simulink model "Main_C0_C3"  (R2023a)
settings: Solver=ode15s  StartTime=0.0  StopTime=1  RelTol=1e-3
model workspace (MAT data in the model file):
  C_IVD = 0.05
  E_IVD1 = 2.1
  E_IVD2 = 2.2
  E_IVD3 = 1.1
  E_IVD4 = 1.7
  E_IVD5 = 3.2
  IVD1 : object (value not decoded)
  IVD2 : object (value not decoded)
  IVD3 : object (value not decoded)
  IVD4 : object (value not decoded)
  IVD5 : object (value not decoded)
  eo_color = [1 0 0]
  io_color = [0 1 0]
  longissimus_color = [1 0 1]
  multifidus_color = [0 1 1]
  muscle_radius = 1
  psoas_color = [0 0 1]
  ra_color = [1 1 0.5]
symbols that are objects in the model workspace (value not decoded): IVD1, IVD2, IVD3, IVD4, IVD5
undefined symbols (not defined in the file or in its folder): AbdFlex, E_TLFflex, IAP_activation_AbdFlex, IAP_Pa, LeftAbdominalMuscleForce, LeftBackMuscleForce, LeftTransverse1MuscleForce, LeftTransverse2MuscleForce, RightAbdominalMuscleForce, RightBackMuscleForce, RightTransverse1MuscleForce, RightTransverse2MuscleForce, TLFflex2, X, Y, Z
libraries: nesl_utility x1235, sm_lib x960, fl_lib x6, simulink_extras x2
(part 8 of 37)

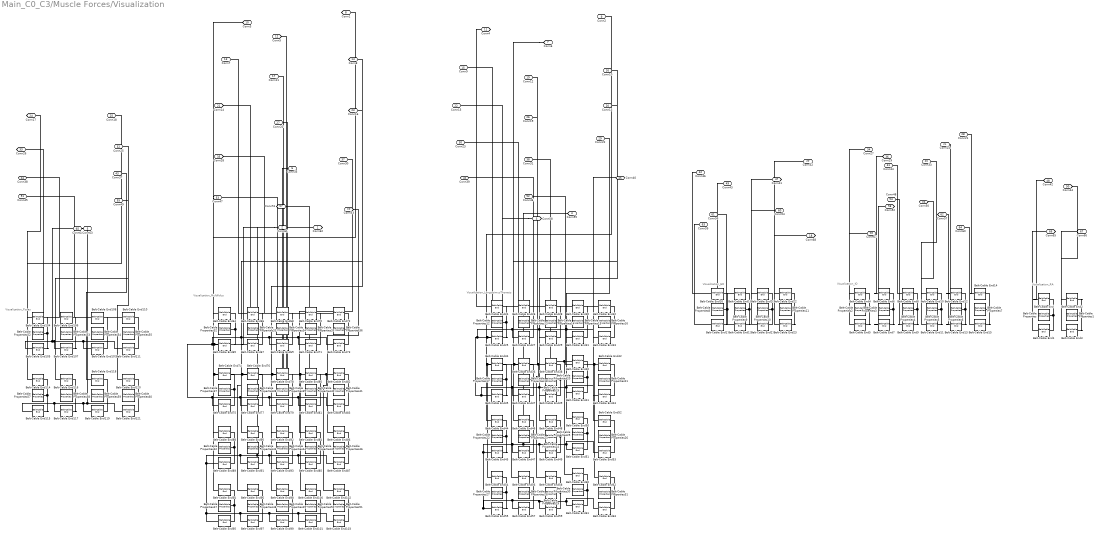
== system Main_C0_C3/Muscle Forces/Visualization ==
  note: Visualization_RA
  note: Visualization_IO
  note: Visualization_EO
  note: Visualization_LongissimusThoracis
  note: Visualization_Multifidus
  note: Visualization_Psoas
  Belt-Cable Properties : sm_lib/Belts and Cables/Belt-Cable Properties  DrumBeltCableAlignment=Unrestricted  GraphicType=PitchLine  GraphicVisPropType=SimpleVisualProperties  GraphicDiffuseColor=[0.302 0.7451 0.9333]  GraphicSpecularColor=[0.5 0.5 0.5 1.0]  GraphicAmbientColor=[0.15 0.15 0.15 1.0]  GraphicEmissiveColor=[0.0 0.0 0.0 1.0]  GraphicShininess=75  GraphicOpacity=1.0
  Belt-Cable Properties1 : sm_lib/Belts and Cables/Belt-Cable Properties  DrumBeltCableAlignment=Unrestricted  GraphicType=PitchLine  GraphicVisPropType=SimpleVisualProperties  GraphicDiffuseColor=[0.302 0.7451 0.9333]  GraphicSpecularColor=[0.5 0.5 0.5 1.0]  GraphicAmbientColor=[0.15 0.15 0.15 1.0]  GraphicEmissiveColor=[0.0 0.0 0.0 1.0]  GraphicShininess=75  GraphicOpacity=1.0
  Belt-Cable Properties{8..11} (4 alike) : sm_lib/Belts and Cables/Belt-Cable Properties  DrumBeltCableAlignment=Unrestricted  GraphicType=PitchLine  GraphicVisPropType=SimpleVisualProperties  GraphicDiffuseColor=[0.851 0.3255 0.09804]  GraphicSpecularColor=[0.5 0.5 0.5 1.0]  GraphicAmbientColor=[0.15 0.15 0.15 1.0]  GraphicEmissiveColor=[0.0 0.0 0.0 1.0]  GraphicShininess=75  GraphicOpacity=1.0
  Belt-Cable Properties{12..31} (20 alike) : sm_lib/Belts and Cables/Belt-Cable Properties  DrumBeltCableAlignment=Unrestricted  GraphicType=PitchLine  GraphicVisPropType=SimpleVisualProperties  GraphicDiffuseColor=[0 0 1]  GraphicSpecularColor=[0.5 0.5 0.5 1.0]  GraphicAmbientColor=[0.15 0.15 0.15 1.0]  GraphicEmissiveColor=[0.0 0.0 0.0 1.0]  GraphicShininess=75  GraphicOpacity=1.0
  Belt-Cable Properties{2..7} (6 alike) : sm_lib/Belts and Cables/Belt-Cable Properties  DrumBeltCableAlignment=Unrestricted  GraphicType=PitchLine  GraphicVisPropType=SimpleVisualProperties  GraphicDiffuseColor=[0.7176 0.2745 1]  GraphicSpecularColor=[0.5 0.5 0.5 1.0]  GraphicAmbientColor=[0.15 0.15 0.15 1.0]  GraphicEmissiveColor=[0.0 0.0 0.0 1.0]  GraphicShininess=75  GraphicOpacity=1.0
  Belt-Cable Properties{32..51} (20 alike) : sm_lib/Belts and Cables/Belt-Cable Properties  DrumBeltCableAlignment=Unrestricted  GraphicType=PitchLine  GraphicVisPropType=SimpleVisualProperties  GraphicDiffuseColor=[0.3922 0.8314 0.07451]  GraphicSpecularColor=[0.5 0.5 0.5 1.0]  GraphicAmbientColor=[0.15 0.15 0.15 1.0]  GraphicEmissiveColor=[0.0 0.0 0.0 1.0]  GraphicShininess=75  GraphicOpacity=1.0
  Belt-Cable Properties{52..55,57..60} (8 alike) : sm_lib/Belts and Cables/Belt-Cable Properties  DrumBeltCableAlignment=Unrestricted  GraphicType=PitchLine  GraphicVisPropType=SimpleVisualProperties  GraphicDiffuseColor=[1 0 0]  GraphicSpecularColor=[0.5 0.5 0.5 1.0]  GraphicAmbientColor=[0.15 0.15 0.15 1.0]  GraphicEmissiveColor=[0.0 0.0 0.0 1.0]  GraphicShininess=75  GraphicOpacity=1.0
  Belt-Cable End{,1..111,114..121} (120 alike) : sm_lib/Belts and Cables/Belt-Cable End
  Conn62 : PMIOPort  Side=Left
  Conn61 : PMIOPort  Port=2  Side=Left
  Conn58 : PMIOPort  Port=3  Side=Left
  Conn55 : PMIOPort  Port=4  Side=Left
  Conn63 : PMIOPort  Port=5  Side=Left
  Conn35 : PMIOPort  Port=6  Side=Left
  Conn6 : PMIOPort  Port=7  Side=Left
  Conn1 : PMIOPort  Port=8  Side=Left
  Conn2 : PMIOPort  Port=9  Side=Left
  Conn3 : PMIOPort  Port=10  Side=Left
  Conn4 : PMIOPort  Port=11  Side=Left
  Conn5 : PMIOPort  Port=12  Side=Left
  Conn7 : PMIOPort  Port=13  Side=Left
  Conn8 : PMIOPort  Port=14  Side=Left
  Conn9 : PMIOPort  Port=15  Side=Left
  Conn10 : PMIOPort  Port=16  Side=Left
  Conn11 : PMIOPort  Port=17  Side=Left
  Conn68 : PMIOPort  Port=18  Side=Left
  Conn12 : PMIOPort  Port=19  Side=Left
  Conn13 : PMIOPort  Port=20  Side=Left
  Conn14 : PMIOPort  Port=21  Side=Left
  Conn15 : PMIOPort  Port=22  Side=Left
  Conn16 : PMIOPort  Port=23  Side=Left
  Conn17 : PMIOPort  Port=24  Side=Left
  Conn18 : PMIOPort  Port=25  Side=Left
  Conn19 : PMIOPort  Port=26  Side=Left
  Conn20 : PMIOPort  Port=27  Side=Left
  Conn21 : PMIOPort  Port=28  Side=Left
  Conn22 : PMIOPort  Port=29  Side=Left
  Conn23 : PMIOPort  Port=30  Side=Left
  Conn24 : PMIOPort  Port=31  Side=Left
  Conn25 : PMIOPort  Port=32  Side=Left
  Conn26 : PMIOPort  Port=33  Side=Left
  Conn27 : PMIOPort  Port=34  Side=Left
  Conn28 : PMIOPort  Port=35  Side=Left
  Conn29 : PMIOPort  Port=36  Side=Left
  Conn30 : PMIOPort  Port=37  Side=Left
  Conn31 : PMIOPort  Port=38  Side=Left
  Conn32 : PMIOPort  Port=39  Side=Left
  Conn33 : PMIOPort  Port=40  Side=Left
  Conn34 : PMIOPort  Port=41  Side=Left
  Conn36 : PMIOPort  Port=42  Side=Left
  Conn37 : PMIOPort  Port=43  Side=Left
  Conn38 : PMIOPort  Port=44  Side=Left
  Conn39 : PMIOPort  Port=45  Side=Left
  Conn40 : PMIOPort  Port=46  Side=Left
  Conn41 : PMIOPort  Port=47  Side=Left
  Conn42 : PMIOPort  Port=48  Side=Left
  Conn43 : PMIOPort  Port=49  Side=Left
  Conn44 : PMIOPort  Port=50  Side=Left
  Conn45 : PMIOPort  Port=51  Side=Left
  Conn46 : PMIOPort  Port=52  Side=Left
  Conn47 : PMIOPort  Port=53  Side=Left
  Conn48 : PMIOPort  Port=54  Side=Left
  Conn49 : PMIOPort  Port=55  Side=Left
  Conn50 : PMIOPort  Port=56  Side=Left
  Conn51 : PMIOPort  Port=57  Side=Left
  Conn52 : PMIOPort  Port=58  Side=Left
  Conn53 : PMIOPort  Port=59  Side=Left
  Conn54 : PMIOPort  Port=60  Side=Left
  Conn56 : PMIOPort  Port=61  Side=Left
  Conn57 : PMIOPort  Port=62  Side=Left
  Conn59 : PMIOPort  Port=63  Side=Left
  Conn60 : PMIOPort  Port=64  Side=Left
  Conn64 : PMIOPort  Port=65  Side=Left
  Conn65 : PMIOPort  Port=66  Side=Left
  Conn66 : PMIOPort  Port=67  Side=Left
  Conn67 : PMIOPort  Port=68  Side=Left
  connections:
  Belt-Cable End64/LConn1 -- Conn3/RConn1
  Belt-Cable End1/LConn1 -- Conn65/RConn1
  Belt-Cable End24/LConn1 -- Conn4/RConn1
  Belt-Cable End28/LConn1 -- Conn15/RConn1
  Belt-Cable End68/LConn1 -- Conn14/RConn1
  Belt-Cable End32/LConn1 -- Conn39/RConn1
  Belt-Cable End48/LConn1 -- Conn13/RConn1
  Belt-Cable End70/LConn1 -- Conn28/RConn1
  Belt-Cable End4/LConn1 -- Conn27/RConn1
  Belt-Cable End13/LConn1 -- Conn57/RConn1
  Belt-Cable End5/LConn1 -- Conn67/RConn1
  Belt-Cable End11/LConn1 -- Conn50/RConn1
  Belt-Cable End9/LConn1 -- Conn48/RConn1
  Belt-Cable End108/LConn1 -- Conn38/RConn1
  Belt-Cable End110/LConn1 -- Conn45/RConn1
  Belt-Cable End52/LConn1 -- Conn40/RConn1
  Belt-Cable End120/LConn1 -- Conn49/RConn1
  Belt-Cable End2/LConn1 -- Conn44/RConn1
  Belt-Cable End22/LConn1 -- Conn32/RConn1
  Belt-Cable End20/LConn1 -- Conn41/RConn1
  Belt-Cable End18/LConn1 -- Conn43/RConn1
  Belt-Cable End19/LConn1 -- Conn56/RConn1
  Belt-Cable End16/LConn1 -- Conn36/RConn1
  Belt-Cable End104/LConn1 -- Conn17/RConn1
  Belt-Cable End116/LConn1 -- Conn25/RConn1
  Belt-Cable Properties15/LConn1 -- Belt-Cable End31/RConn1 -- Belt-Cable End30/RConn1
  Belt-Cable End12/LConn1 -- Conn24/RConn1
  Belt-Cable Properties12/LConn1 -- Belt-Cable End25/RConn1 -- Belt-Cable End24/RConn1
  Belt-Cable End46/LConn1 -- Conn10/RConn1
  Belt-Cable End3/LConn1 -- Conn66/RConn1
  Belt-Cable End114/LConn1 -- Conn18/RConn1
  Conn5/RConn1 -- Belt-Cable End74/LConn1 -- Belt-Cable End94/LConn1
  Belt-Cable End72/LConn1 -- Conn47/RConn1
  Belt-Cable End/LConn1 -- Conn42/RConn1
  Belt-Cable End90/LConn1 -- Conn8/RConn1
  Belt-Cable End23/LConn1 -- Conn68/RConn1
  Belt-Cable Properties59/LConn1 -- Belt-Cable End119/RConn1 -- Belt-Cable End118/RConn1
  Belt-Cable End44/LConn1 -- Conn2/RConn1
  Belt-Cable Properties37/LConn1 -- Belt-Cable End75/RConn1 -- Belt-Cable End74/RConn1
  Belt-Cable End10/LConn1 -- Conn33/RConn1
  Belt-Cable Properties53/LConn1 -- Belt-Cable End107/RConn1 -- Belt-Cable End106/RConn1
  Belt-Cable End30/LConn1 -- Conn23/RConn1
  Conn6/RConn1 -- Belt-Cable End34/LConn1 -- Belt-Cable End54/LConn1
  Belt-Cable End14/LConn1 -- Conn21/RConn1
  Belt-Cable End88/LConn1 -- Conn1/RConn1
  Belt-Cable End86/LConn1 -- Conn53/RConn1
  Belt-Cable Properties52/LConn1 -- Belt-Cable End105/RConn1 -- Belt-Cable End104/RConn1
  Belt-Cable Properties5/LConn1 -- Belt-Cable End11/RConn1 -- Belt-Cable End10/RConn1
  Belt-Cable End117/LConn1 -- Belt-Cable End119/LConn1 -- Conn64/RConn1 -- Belt-Cable End121/LConn1 -- Belt-Cable End115/LConn1
  Belt-Cable Properties38/LConn1 -- Belt-Cable End77/RConn1 -- Belt-Cable End76/RConn1
  Belt-Cable Properties35/LConn1 -- Belt-Cable End71/RConn1 -- Belt-Cable End70/RConn1
  Belt-Cable End8/LConn1 -- Conn34/RConn1
  Belt-Cable End15/LConn1 -- Conn60/RConn1
  Belt-Cable Properties33/LConn1 -- Belt-Cable End67/RConn1 -- Belt-Cable End66/RConn1
  Belt-Cable Properties21/LConn1 -- Belt-Cable End43/RConn1 -- Belt-Cable End42/RConn1
  Belt-Cable Properties41/LConn1 -- Belt-Cable End83/RConn1 -- Belt-Cable End82/RConn1
  Belt-Cable Properties58/LConn1 -- Belt-Cable End117/RConn1 -- Belt-Cable End116/RConn1
  Conn20/RConn1 -- Belt-Cable End78/LConn1 -- Belt-Cable End98/LConn1
  Belt-Cable Properties2/LConn1 -- Belt-Cable End5/RConn1 -- Belt-Cable End4/RConn1
  Belt-Cable End66/LConn1 -- Conn7/RConn1
  Belt-Cable Properties48/LConn1 -- Belt-Cable End97/RConn1 -- Belt-Cable End96/RConn1
  Belt-Cable Properties51/LConn1 -- Belt-Cable End103/RConn1 -- Belt-Cable End102/RConn1
  Belt-Cable Properties23/LConn1 -- Belt-Cable End47/RConn1 -- Belt-Cable End46/RConn1
  Belt-Cable Properties40/LConn1 -- Belt-Cable End81/RConn1 -- Belt-Cable End80/RConn1
  Belt-Cable Properties36/LConn1 -- Belt-Cable End73/RConn1 -- Belt-Cable End72/RConn1
  Belt-Cable Properties46/LConn1 -- Belt-Cable End87/RConn1 -- Belt-Cable End86/RConn1
  Belt-Cable End6/LConn1 -- Conn29/RConn1
  Belt-Cable End26/LConn1 -- Conn9/RConn1
  Belt-Cable Properties11/LConn1 -- Belt-Cable End23/RConn1 -- Belt-Cable End22/RConn1
  Belt-Cable Properties24/LConn1 -- Belt-Cable End49/RConn1 -- Belt-Cable End48/RConn1
  Belt-Cable End/RConn1 -- Belt-Cable Properties/LConn1 -- Belt-Cable End1/RConn1
  Belt-Cable End38/LConn1 -- Conn19/RConn1 -- Belt-Cable End58/LConn1
  Belt-Cable End106/LConn1 -- Conn26/RConn1
  Belt-Cable Properties10/LConn1 -- Belt-Cable End21/RConn1 -- Belt-Cable End20/RConn1
  Belt-Cable Properties47/LConn1 -- Belt-Cable End95/RConn1 -- Belt-Cable End94/RConn1
  Belt-Cable End118/LConn1 -- Conn37/RConn1
  Belt-Cable End17/LConn1 -- Conn59/RConn1
  Belt-Cable Properties39/LConn1 -- Belt-Cable End79/RConn1 -- Belt-Cable End78/RConn1
  Belt-Cable Properties45/LConn1 -- Belt-Cable End85/RConn1 -- Belt-Cable End84/RConn1
  Belt-Cable Properties20/LConn1 -- Belt-Cable End41/RConn1 -- Belt-Cable End40/RConn1
  Belt-Cable Properties8/LConn1 -- Belt-Cable End17/RConn1 -- Belt-Cable End16/RConn1
  Belt-Cable Properties49/LConn1 -- Belt-Cable End99/RConn1 -- Belt-Cable End98/RConn1
  Belt-Cable Properties6/LConn1 -- Belt-Cable End13/RConn1 -- Belt-Cable End12/RConn1
  Belt-Cable Properties28/LConn1 -- Belt-Cable End57/RConn1 -- Belt-Cable End56/RConn1
  Belt-Cable Properties27/LConn1 -- Belt-Cable End55/RConn1 -- Belt-Cable End54/RConn1
  Belt-Cable End7/LConn1 -- Conn52/RConn1
  Belt-Cable End60/LConn1 -- Conn31/RConn1 -- Belt-Cable End40/LConn1
  Belt-Cable Properties4/LConn1 -- Belt-Cable End9/RConn1 -- Belt-Cable End8/RConn1
  Belt-Cable Properties44/LConn1 -- Belt-Cable End93/RConn1 -- Belt-Cable End92/RConn1
  Belt-Cable Properties57/LConn1 -- Belt-Cable End115/RConn1 -- Belt-Cable End114/RConn1
  Conn12/RConn1 -- Belt-Cable End36/LConn1 -- Belt-Cable End56/LConn1
  Belt-Cable Properties54/LConn1 -- Belt-Cable End109/RConn1 -- Belt-Cable End108/RConn1
  Belt-Cable End21/LConn1 -- Conn54/RConn1
  Belt-Cable Properties3/LConn1 -- Belt-Cable End7/RConn1 -- Belt-Cable End6/RConn1
  Belt-Cable Properties55/LConn1 -- Belt-Cable End111/RConn1 -- Belt-Cable End110/RConn1
  Belt-Cable Properties34/LConn1 -- Belt-Cable End69/RConn1 -- Belt-Cable End68/RConn1
  Belt-Cable Properties26/LConn1 -- Belt-Cable End53/RConn1 -- Belt-Cable End52/RConn1
  Belt-Cable Properties18/LConn1 -- Belt-Cable End37/RConn1 -- Belt-Cable End36/RConn1
  Belt-Cable Properties29/LConn1 -- Belt-Cable End59/RConn1 -- Belt-Cable End58/RConn1
  Belt-Cable Properties22/LConn1 -- Belt-Cable End45/RConn1 -- Belt-Cable End44/RConn1
  Belt-Cable End92/LConn1 -- Conn16/RConn1
  Belt-Cable Properties17/LConn1 -- Belt-Cable End35/RConn1 -- Belt-Cable End34/RConn1
  Belt-Cable Properties14/LConn1 -- Belt-Cable End29/RConn1 -- Belt-Cable End28/RConn1
  Belt-Cable Properties50/LConn1 -- Belt-Cable End101/RConn1 -- Belt-Cable End100/RConn1
  Belt-Cable Properties31/LConn1 -- Belt-Cable End63/RConn1 -- Belt-Cable End62/RConn1
  Belt-Cable End76/LConn1 -- Conn11/RConn1 -- Belt-Cable End96/LConn1
  Belt-Cable Properties7/LConn1 -- Belt-Cable End15/RConn1 -- Belt-Cable End14/RConn1
  Conn61/RConn1 -- Belt-Cable End65/LConn1 -- Belt-Cable End75/LConn1 -- Belt-Cable End77/LConn1 -- Belt-Cable End79/LConn1 -- Belt-Cable End83/LConn1 -- Belt-Cable End81/LConn1 -- Belt-Cable End67/LConn1 -- Belt-Cable End69/LConn1 -- Belt-Cable End73/LConn1 -- Belt-Cable End71/LConn1
  Belt-Cable Properties42/LConn1 -- Belt-Cable End89/RConn1 -- Belt-Cable End88/RConn1
  Belt-Cable End2/RConn1 -- Belt-Cable End3/RConn1 -- Belt-Cable Properties1/LConn1
  Belt-Cable End95/LConn1 -- Belt-Cable End89/LConn1 -- Belt-Cable End91/LConn1 -- Conn62/RConn1 -- Belt-Cable End93/LConn1 -- Belt-Cable End87/LConn1 -- Belt-Cable End85/LConn1 -- Belt-Cable End97/LConn1 -- Belt-Cable End103/LConn1 -- Belt-Cable End101/LConn1 -- Belt-Cable End99/LConn1
  Belt-Cable End65/RConn1 -- Belt-Cable End64/RConn1 -- Belt-Cable Properties32/LConn1
  Belt-Cable End84/LConn1 -- Conn30/RConn1
  Belt-Cable Properties16/LConn1 -- Belt-Cable End33/RConn1 -- Belt-Cable End32/RConn1
  Belt-Cable Properties30/LConn1 -- Belt-Cable End61/RConn1 -- Belt-Cable End60/RConn1
  Conn63/RConn1 -- Belt-Cable End105/LConn1 -- Belt-Cable End107/LConn1 -- Belt-Cable End109/LConn1 -- Belt-Cable End111/LConn1
  Belt-Cable Properties9/LConn1 -- Belt-Cable End19/RConn1 -- Belt-Cable End18/RConn1
  Belt-Cable Properties60/LConn1 -- Belt-Cable End121/RConn1 -- Belt-Cable End120/RConn1
  Belt-Cable End80/LConn1 -- Conn35/RConn1 -- Belt-Cable End100/LConn1
  Belt-Cable Properties25/LConn1 -- Belt-Cable End51/RConn1 -- Belt-Cable End50/RConn1
  Conn58/RConn1 -- Belt-Cable End27/LConn1 -- Belt-Cable End29/LConn1 -- Belt-Cable End31/LConn1 -- Belt-Cable End33/LConn1 -- Belt-Cable End35/LConn1 -- Belt-Cable End37/LConn1 -- Belt-Cable End39/LConn1 -- Belt-Cable End43/LConn1 -- Belt-Cable End41/LConn1 -- Belt-Cable End25/LConn1
  Belt-Cable Properties43/LConn1 -- Belt-Cable End91/RConn1 -- Belt-Cable End90/RConn1
  Conn51/RConn1 -- Belt-Cable End82/LConn1 -- Belt-Cable End102/LConn1
  Belt-Cable End42/LConn1 -- Conn46/RConn1 -- Belt-Cable End62/LConn1
  Belt-Cable Properties19/LConn1 -- Belt-Cable End39/RConn1 -- Belt-Cable End38/RConn1
  Belt-Cable End59/LConn1 -- Belt-Cable End55/LConn1 -- Belt-Cable End45/LConn1 -- Belt-Cable End47/LConn1 -- Conn55/RConn1 -- Belt-Cable End49/LConn1 -- Belt-Cable End53/LConn1 -- Belt-Cable End51/LConn1 -- Belt-Cable End57/LConn1 -- Belt-Cable End63/LConn1 -- Belt-Cable End61/LConn1
  Belt-Cable End50/LConn1 -- Conn22/RConn1
  Belt-Cable Properties13/LConn1 -- Belt-Cable End27/RConn1 -- Belt-Cable End26/RConn1

== system Main_C0_C3/Supraspinous Ligaments/SSL Visualization ==
  Ligament1 : Subsystem
  Ligament2 : Subsystem
  Ligament3 : Subsystem
  Ligament4 : Subsystem
  Ligament6 : Subsystem
  MuscleEnd2 : PMIOPort  Side=Right
  MuscleEnd1 : PMIOPort  Port=2  Side=Right
  MuscleEnd3 : PMIOPort  Port=3  Side=Right
  MuscleEnd4 : PMIOPort  Port=4  Side=Right
  MuscleEnd5 : PMIOPort  Port=5  Side=Right
  MuscleEnd6 : PMIOPort  Port=6  Side=Right
  MuscleEnd7 : PMIOPort  Port=7  Side=Right
  MuscleEnd8 : PMIOPort  Port=8  Side=Right
  MuscleEnd9 : PMIOPort  Port=9  Side=Right
  MuscleEnd10 : PMIOPort  Port=10  Side=Right
  R : PMIOPort  Port=11  Side=Left
  connections:
  Ligament6/RConn1 -- MuscleEnd10/RConn1
  Ligament4/RConn2 -- MuscleEnd1/RConn1
  Ligament1/RConn2 -- MuscleEnd5/RConn1
  Ligament6/RConn2 -- MuscleEnd9/RConn1
  Ligament4/RConn1 -- MuscleEnd4/RConn1
  Ligament2/RConn1 -- MuscleEnd8/RConn1
  Ligament1/RConn1 -- MuscleEnd7/RConn1
  Ligament2/RConn2 -- MuscleEnd6/RConn1
  Ligament3/RConn1 -- MuscleEnd3/RConn1
  R/RConn1 -- Ligament1/RConn3 -- Ligament2/RConn3 -- Ligament3/RConn3 -- Ligament4/RConn3 -- Ligament6/RConn3
  Ligament3/RConn2 -- MuscleEnd2/RConn1

== system Main_C0_C3/Supraspinous Ligaments/Visualization ==
  Belt-Cable Properties{1..4,55} (5 alike) : sm_lib/Belts and Cables/Belt-Cable Properties  DrumBeltCableAlignment=Unrestricted  GraphicType=PitchLine  GraphicVisPropType=SimpleVisualProperties  GraphicDiffuseColor=[0.6353 0.07843 0.1843]  GraphicSpecularColor=[0.5 0.5 0.5 1.0]  GraphicAmbientColor=[0.15 0.15 0.15 1.0]  GraphicEmissiveColor=[0.0 0.0 0.0 1.0]  GraphicShininess=75  GraphicOpacity=1.0
  Belt-Cable End{1..8,110..111} (10 alike) : sm_lib/Belts and Cables/Belt-Cable End
  Conn1 : PMIOPort  Side=Left
  Conn2 : PMIOPort  Port=2  Side=Left
  Conn3 : PMIOPort  Port=3  Side=Left
  Conn4 : PMIOPort  Port=4  Side=Left
  Conn5 : PMIOPort  Port=5  Side=Left
  Conn6 : PMIOPort  Port=6  Side=Left
  Conn7 : PMIOPort  Port=7  Side=Left
  Conn8 : PMIOPort  Port=8  Side=Left
  Conn9 : PMIOPort  Port=9  Side=Left
  Conn10 : PMIOPort  Port=10  Side=Left
  connections:
  Belt-Cable End7/LConn1 -- Conn1/RConn1
  Belt-Cable End111/LConn1 -- Conn9/RConn1
  Belt-Cable End4/LConn1 -- Conn2/RConn1
  Belt-Cable End6/LConn1 -- Conn6/RConn1
  Belt-Cable End110/LConn1 -- Conn5/RConn1
  Belt-Cable End5/LConn1 -- Conn7/RConn1
  Belt-Cable End1/LConn1 -- Conn3/RConn1
  Belt-Cable End8/LConn1 -- Conn10/RConn1
  Belt-Cable Properties3/LConn1 -- Belt-Cable End5/RConn1 -- Belt-Cable End4/RConn1
  Belt-Cable End3/RConn1 -- Belt-Cable End6/RConn1 -- Belt-Cable Properties2/LConn1
  Belt-Cable End2/RConn1 -- Belt-Cable End1/RConn1 -- Belt-Cable Properties1/LConn1
  Belt-Cable End2/LConn1 -- Conn8/RConn1
  Belt-Cable Properties4/LConn1 -- Belt-Cable End8/RConn1 -- Belt-Cable End7/RConn1
  Belt-Cable End3/LConn1 -- Conn4/RConn1
  Belt-Cable End110/RConn1 -- Belt-Cable End111/RConn1 -- Belt-Cable Properties55/LConn1

== system Main_C0_C3/TLF Flex/Latissimus Dorsi ==
  In1 : Inport
  In2 : Inport  Port=2
  Gain : Gain  Gain=-0.3333
  Gain1 : Gain  Gain=-0.3333
  Internal Force{,1..5} (6 alike) : sm_lib/Forces and Torques/Internal Force
  Left Clavicle : sm_lib/Body Elements/File Solid  ExtGeomFileName=C:\Users\siril\OneDrive\Desktop\TIM-Control\Matlab\Simscape models\Reduced Order Model\CAD\Left_Clavicle.step  UnitType=FromFile  ExtGeomFileUnits=m  StepReaderType=HEX  ExportConvexHullGeometry=off  InertiaType=CalculateFromGeometry  Mass=1  MassUnits=kg  CenterOfMass=[0 0 0]  CenterOfMassUnits=m  MomentsOfInertia=[1 1 1]  MomentsOfInertiaUnits=kg*m^2  ProductsOfInertia=[0 0 0]  ProductsOfInertiaUnits=kg*m^2  BasedOnType=Density  Density=0.18  DensityUnits=g/cm^3  DoExposeReferenceFrame=off  SerializedFrames=<Frames><Frame><Id>Frame1</Id><Value><Name>To Left Lats</Name><Origin><Source>GeometricFeature</Source><FeatureName>planar surface 1150</FeatureName></Origin><PrimaryAxis><DefinedDirection>+Z</DefinedDirection><Source>ReferenceFrame</Source><SourceDirection>+Z</SourceDirection><FeatureName></FeatureName></PrimaryAxis><SecondaryAxis><DefinedDirection>+X</DefinedDirection><Source>ReferenceFrame</Source><SourceDirection>+X</SourceDirection><FeatureName></FeatureName></SecondaryAxis></Value></Frame><Frame><Id>Frame2</Id><Value><Name>To Left T Spine</Name><Origin><Source>GeometricFeature</Source><FeatureName>point 146</FeatureName></Origin><PrimaryAxis><DefinedDirection>+Z</DefinedDirection><Source>ReferenceFrame</Source><SourceDirection>+Z</SourceDirection><FeatureName></FeatureName></PrimaryAxis><SecondaryAxis><DefinedDirection>+X</DefinedDirection><Source>ReferenceFrame</Source><SourceDirection>+X</SourceDirection><FeatureName></FeatureName></SecondaryAxis></Value></Frame></Frames>  GraphicType=None  MarkerShape=Sphere  MarkerSize=10  GraphicVisPropType=SimpleVisualProperties  GraphicDiffuseColor=[0.8901961 0.85490197 0.7882353]  GraphicSpecularColor=[0.5 0.5 0.5 1.0]  GraphicAmbientColor=[0.15 0.15 0.15 1.0]  GraphicEmissiveColor=[0.0 0.0 0.0 1.0]  GraphicShininess=75  GraphicOpacity=0.5
  Right Clavicle : sm_lib/Body Elements/File Solid  ExtGeomFileName=C:\Users\siril\OneDrive\Desktop\TIM-Control\Matlab\Simscape models\CAD - with COM\SymmetricModel\draft7\Right Hand\Clavicle.step  UnitType=FromFile  ExtGeomFileUnits=m  StepReaderType=HEX  ExportConvexHullGeometry=off  InertiaType=CalculateFromGeometry  Mass=1  MassUnits=kg  CenterOfMass=[0 0 0]  CenterOfMassUnits=m  MomentsOfInertia=[1 1 1]  MomentsOfInertiaUnits=kg*m^2  ProductsOfInertia=[0 0 0]  ProductsOfInertiaUnits=kg*m^2  BasedOnType=Density  Density=0.18  DensityUnits=g/cm^3  DoExposeReferenceFrame=off  SerializedFrames=<Frames><Frame><Id>Frame1</Id><Value><Name>To Right Lats</Name><Origin><Source>GeometricFeature</Source><FeatureName>planar surface 1150</FeatureName></Origin><PrimaryAxis><DefinedDirection>+Z</DefinedDirection><Source>ReferenceFrame</Source><SourceDirection>+Z</SourceDirection><FeatureName></FeatureName></PrimaryAxis><SecondaryAxis><DefinedDirection>+X</DefinedDirection><Source>ReferenceFrame</Source><SourceDirection>+X</SourceDirection><FeatureName></FeatureName></SecondaryAxis></Value></Frame><Frame><Id>Frame2</Id><Value><Name>To Right T Spine</Name><Origin><Source>GeometricFeature</Source><FeatureName>point 146</FeatureName></Origin><PrimaryAxis><DefinedDirection>+Z</DefinedDirection><Source>ReferenceFrame</Source><SourceDirection>+Z</SourceDirection><FeatureName></FeatureName></PrimaryAxis><SecondaryAxis><DefinedDirection>+X</DefinedDirection><Source>ReferenceFrame</Source><SourceDirection>+X</SourceDirection><FeatureName></FeatureName></SecondaryAxis></Value></Frame></Frames>  GraphicType=None  MarkerShape=Sphere  MarkerSize=10  GraphicVisPropType=SimpleVisualProperties  GraphicDiffuseColor=[0.8901961 0.85490197 0.7882353]  GraphicSpecularColor=[0.5 0.5 0.5 1.0]  GraphicAmbientColor=[0.15 0.15 0.15 1.0]  GraphicEmissiveColor=[0.0 0.0 0.0 1.0]  GraphicShininess=75  GraphicOpacity=0.5
  Simulink-PS Converter{,1..5} (6 alike) : nesl_utility/Simulink-PS Converter  PhysicalDomain=network_engine_domain  SubClassName=ps_input  LeftPortType=input  RightPortType=output  PseudoPeriodic=off  Frequencies=[]  NoiseDistribution=none  NoiseParameters=[]  Unit=1  AffineConversion=off  FilteringAndDerivatives=provide  SimscapeFilterOrder=1  InputFilterTimeConstant=0.001  UdotUserProvided=0
  WrappedMuscle1 : Subsystem
  WrappedMuscle2 : Subsystem
  WrappedMuscle3 : Subsystem
  WrappedMuscle4 : Subsystem
  WrappedMuscle5 : Subsystem
  WrappedMuscle7 : Subsystem
  Conn1 : PMIOPort  Side=Right
  MuscleEnd2 : PMIOPort  Port=2  Side=Right
  MuscleEnd1 : PMIOPort  Port=3  Side=Left
  Conn4 : PMIOPort  Port=4  Side=Right
  MuscleEnd3 : PMIOPort  Port=5  Side=Left
  Conn6 : PMIOPort  Port=6  Side=Right
  Conn7 : PMIOPort  Port=7  Side=Left
  Conn8 : PMIOPort  Port=8  Side=Left
  Conn9 : PMIOPort  Port=9  Side=Left
  Wrap1 : PMIOPort  Port=10  Side=Right
  Wrap2 : PMIOPort  Port=11  Side=Right
  Conn12 : PMIOPort  Port=12  Side=Left
  Conn13 : PMIOPort  Port=13  Side=Right
  Conn14 : PMIOPort  Port=14  Side=Left
  Wrap3 : PMIOPort  Port=15  Side=Right
  Wrap4 : PMIOPort  Port=16  Side=Right
  Wrap5 : PMIOPort  Port=17  Side=Right
  Conn18 : PMIOPort  Port=18  Side=Right
  wires:
  Gain/1 -> Simulink-PS Converter3/1, Simulink-PS Converter4/1, Simulink-PS Converter5/1
  In2/1 -> Gain/1
  Gain1/1 -> Simulink-PS Converter2/1, Simulink-PS Converter1/1, Simulink-PS Converter/1
  In1/1 -> Gain1/1
  connections:
  WrappedMuscle4/RConn2 -- Wrap3/RConn1
  WrappedMuscle2/RConn2 -- Wrap1/RConn1
  Conn1/RConn1 -- Right Clavicle/RConn1
  WrappedMuscle1/RConn2 -- Wrap4/RConn1
  Internal Force4/LConn1 -- Conn7/RConn1 -- WrappedMuscle5/RConn4
  Internal Force1/RConn1 -- Conn9/RConn1 -- WrappedMuscle4/RConn3
  Simulink-PS Converter5/RConn1 -- Internal Force5/LConn2
  Internal Force2/RConn1 -- Conn8/RConn1 -- WrappedMuscle3/RConn2
  WrappedMuscle5/RConn2 -- Wrap2/RConn1
  WrappedMuscle3/RConn3 -- MuscleEnd3/RConn1 -- Internal Force2/LConn1
  Conn4/RConn1 -- Internal Force3/LConn1 -- WrappedMuscle2/RConn4
  Internal Force2/LConn2 -- Simulink-PS Converter2/RConn1
  Internal Force5/RConn1 -- Conn14/RConn1 -- WrappedMuscle7/RConn2
  Internal Force4/RConn1 -- Conn13/RConn1 -- WrappedMuscle5/RConn3
  Conn18/RConn1 -- Left Clavicle/RConn1
  Internal Force/LConn2 -- Simulink-PS Converter/RConn1
  Wrap5/RConn1 -- WrappedMuscle1/RConn3 -- Internal Force/RConn1
  WrappedMuscle4/RConn4 -- MuscleEnd2/RConn1 -- Internal Force1/LConn1
  Internal Force3/RConn1 -- Conn12/RConn1 -- WrappedMuscle2/RConn3
  Conn6/RConn1 -- Internal Force5/LConn1 -- WrappedMuscle7/RConn3
  Simulink-PS Converter4/RConn1 -- Internal Force4/LConn2
  Left Clavicle/LConn1 -- WrappedMuscle5/RConn1 -- WrappedMuscle7/RConn1 -- WrappedMuscle2/RConn1
  WrappedMuscle1/RConn1 -- WrappedMuscle4/RConn1 -- WrappedMuscle3/RConn1 -- Right Clavicle/LConn1
  WrappedMuscle1/RConn4 -- MuscleEnd1/RConn1 -- Internal Force/LConn1
  Internal Force1/LConn2 -- Simulink-PS Converter1/RConn1
  Simulink-PS Converter3/RConn1 -- Internal Force3/LConn2

== system Main_C0_C3/Interspinous Ligaments/ISL Visualization/Ligament1 ==
  Constant : Constant  Value=0
  Constant1 : Constant  Value=0
  Gimbal Joint : sm_lib/Joints/Gimbal Joint  JointMode=Normal  SenseConstraintForce=off  SenseConstraintForceX=off  SenseConstraintForceY=off  SenseConstraintForceZ=off  SenseConstraintTorque=off  SenseConstraintTorqueX=off  SenseConstraintTorqueY=off  SenseConstraintTorqueZ=off  SenseTotalForce=off  SenseTotalForceX=off  SenseTotalForceY=off  SenseTotalForceZ=off  SenseTotalTorque=off  SenseTotalTorqueX=off  SenseTotalTorqueY=off  SenseTotalTorqueZ=off  CompositeWrenchDir=FollowerOnBase  CompositeWrenchFrame=BaseFrame  RxEquilibriumPosition=0  RxEquilibriumPositionUnits=deg  RxSpringStiffness=0  RxSpringStiffnessUnits=N*m/deg  RxDampingCoefficient=0  RxDampingCoefficientUnits=N*m/(deg/s)  RxTorqueActuationMode=ComputedTorque  RxMotionActuationMode=InputMotion  RxSensePosition=off  RxSenseVelocity=off  RxSenseAcceleration=off  RxSenseTorqueForce=off  RxSenseLowerLimitTorqueForce=off  RxSenseUpperLimitTorqueForce=off  RxLowerLimitSpecify=off  RxLowerLimitBound=-90  RxLowerLimitBoundUnits=deg  RxLowerLimitStiffness=1e4  RxLowerLimitStiffnessUnits=N*m/deg  RxLowerLimitDamping=10  RxLowerLimitDampingUnits=N*m/(deg/s)  RxLowerLimitTransitionRegionWidth=0.1  RxLowerLimitTransitionRegionWidthUnits=deg  RxUpperLimitSpecify=off  RxUpperLimitBound=90  RxUpperLimitBoundUnits=deg  RxUpperLimitStiffness=1e4  RxUpperLimitStiffnessUnits=N*m/deg  RxUpperLimitDamping=10  RxUpperLimitDampingUnits=N*m/(deg/s)  RxUpperLimitTransitionRegionWidth=0.1  RxUpperLimitTransitionRegionWidthUnits=deg  RxPositionTargetSpecify=off  RxPositionTargetPriority=High  RxPositionTargetValue=0  RxPositionTargetValueUnits=deg  RxVelocityTargetSpecify=off  RxVelocityTargetPriority=High  RxVelocityTargetValue=0  RxVelocityTargetValueUnits=deg/s  RyEquilibriumPosition=0  RyEquilibriumPositionUnits=deg  RySpringStiffness=0  RySpringStiffnessUnits=N*m/deg  RyDampingCoefficient=0  RyDampingCoefficientUnits=N*m/(deg/s)  RyTorqueActuationMode=ComputedTorque  RyMotionActuationMode=InputMotion  RySensePosition=off  RySenseVelocity=off  RySenseAcceleration=off  RySenseTorqueForce=off  RySenseLowerLimitTorqueForce=off  RySenseUpperLimitTorqueForce=off  RyLowerLimitSpecify=off  RyLowerLimitBound=-90  RyLowerLimitBoundUnits=deg  RyLowerLimitStiffness=1e4  RyLowerLimitStiffnessUnits=N*m/deg  RyLowerLimitDamping=10  RyLowerLimitDampingUnits=N*m/(deg/s)  RyLowerLimitTransitionRegionWidth=0.1  RyLowerLimitTransitionRegionWidthUnits=deg  RyUpperLimitSpecify=off  RyUpperLimitBound=90  RyUpperLimitBoundUnits=deg  RyUpperLimitStiffness=1e4  RyUpperLimitStiffnessUnits=N*m/deg  RyUpperLimitDamping=10  RyUpperLimitDampingUnits=N*m/(deg/s)  RyUpperLimitTransitionRegionWidth=0.1  RyUpperLimitTransitionRegionWidthUnits=deg  RyPositionTargetSpecify=off  RyPositionTargetPriority=High  RyPositionTargetValue=0  RyPositionTargetValueUnits=deg  RyVelocityTargetSpecify=off  RyVelocityTargetPriority=High  RyVelocityTargetValue=0  RyVelocityTargetValueUnits=deg/s  RzEquilibriumPosition=0  RzEquilibriumPositionUnits=deg  RzSpringStiffness=0  RzSpringStiffnessUnits=N*m/deg  RzDampingCoefficient=0  RzDampingCoefficientUnits=N*m/(deg/s)  RzTorqueActuationMode=ComputedTorque  RzMotionActuationMode=InputMotion  RzSensePosition=off  RzSenseVelocity=off  RzSenseAcceleration=off  RzSenseTorqueForce=off  RzSenseLowerLimitTorqueForce=off  RzSenseUpperLimitTorqueForce=off  RzLowerLimitSpecify=off  RzLowerLimitBound=-90  RzLowerLimitBoundUnits=deg  RzLowerLimitStiffness=1e4  RzLowerLimitStiffnessUnits=N*m/deg  RzLowerLimitDamping=10  RzLowerLimitDampingUnits=N*m/(deg/s)  RzLowerLimitTransitionRegionWidth=0.1  RzLowerLimitTransitionRegionWidthUnits=deg  RzUpperLimitSpecify=off  RzUpperLimitBound=90  RzUpperLimitBoundUnits=deg  RzUpperLimitStiffness=1e4  RzUpperLimitStiffnessUnits=N*m/deg  RzUpperLimitDamping=10  RzUpperLimitDampingUnits=N*m/(deg/s)  RzUpperLimitTransitionRegionWidth=0.1  RzUpperLimitTransitionRegionWidthUnits=deg  RzPositionTargetSpecify=off  RzPositionTargetPriority=High  RzPositionTargetValue=0  RzPositionTargetValueUnits=deg  RzVelocityTargetSpecify=off  RzVelocityTargetPriority=High  RzVelocityTargetValue=0  RzVelocityTargetValueUnits=deg/s
  MATLAB Function2 : MATLAB Function  TreatAsAtomicUnit=on
  PS-Simulink Converter{,6..7,11..13} (6 alike) : nesl_utility/PS-Simulink Converter  PhysicalDomain=network_engine_domain  SubClassName=ps_output  LeftPortType=input  RightPortType=output  PseudoPeriodic=off  Frequencies=[]  VectorFormat=inherit  Unit=inherit  AffineConversion=off
  Simulink-PS Converter : nesl_utility/Simulink-PS Converter  PhysicalDomain=network_engine_domain  SubClassName=ps_input  LeftPortType=input  RightPortType=output  PseudoPeriodic=off  Frequencies=[]  NoiseDistribution=none  NoiseParameters=[]  Unit=m  AffineConversion=off  FilteringAndDerivatives=provide  SimscapeFilterOrder=1  InputFilterTimeConstant=0.001  UdotUserProvided=0
  Simulink-PS Converter10 : nesl_utility/Simulink-PS Converter  PhysicalDomain=network_engine_domain  SubClassName=ps_input  LeftPortType=input  RightPortType=output  PseudoPeriodic=off  Frequencies=[]  NoiseDistribution=none  NoiseParameters=[]  Unit=1  AffineConversion=off  FilteringAndDerivatives=provide  SimscapeFilterOrder=2  InputFilterTimeConstant=0.001  UdotUserProvided=2
  Simulink-PS Converter11 : nesl_utility/Simulink-PS Converter  PhysicalDomain=network_engine_domain  SubClassName=ps_input  LeftPortType=input  RightPortType=output  PseudoPeriodic=off  Frequencies=[]  NoiseDistribution=none  NoiseParameters=[]  Unit=1  AffineConversion=off  FilteringAndDerivatives=provide  SimscapeFilterOrder=2  InputFilterTimeConstant=0.001  UdotUserProvided=2
  Simulink-PS Converter9 : nesl_utility/Simulink-PS Converter  PhysicalDomain=network_engine_domain  SubClassName=ps_input  LeftPortType=input  RightPortType=output  PseudoPeriodic=off  Frequencies=[]  NoiseDistribution=none  NoiseParameters=[]  Unit=1  AffineConversion=on  FilteringAndDerivatives=provide  SimscapeFilterOrder=2  InputFilterTimeConstant=0.1  UdotUserProvided=2
  Transform Sensor : sm_lib/Frames and Transforms/Transform Sensor  MeasurementFrame=Base  RotationSequence=XYZ  SenseAngle=off  SenseAxis=off  SenseQ=off  SenseR=off  SenseRotationSequence=off  SenseOmegaX=off  SenseOmegaY=off  SenseOmegaZ=off  SenseQDot=off  SenseRDot=off  SenseRotationSequenceDot=off  SenseAlphaX=off  SenseAlphaY=off  SenseAlphaZ=off  SenseQDDot=off  SenseRDDot=off  SenseX=on  SenseY=on  SenseZ=on  SenseRad=off  SenseAzim=off  SenseDist=off  SenseInc=off  SenseXDot=off  SenseYDot=off  SenseZDot=off  SenseRadDot=off  SenseAzimDot=off  SenseDistDot=off  SenseIncDot=off  SenseXDDot=off  SenseYDDot=off  SenseZDDot=off  SenseRadDDot=off  SenseAzimDDot=off  SenseDistDDot=off  SenseIncDDot=off
  Transform Sensor1 : sm_lib/Frames and Transforms/Transform Sensor  MeasurementFrame=Base  RotationSequence=XYZ  SenseAngle=off  SenseAxis=off  SenseQ=off  SenseR=off  SenseRotationSequence=off  SenseOmegaX=off  SenseOmegaY=off  SenseOmegaZ=off  SenseQDot=off  SenseRDot=off  SenseRotationSequenceDot=off  SenseAlphaX=off  SenseAlphaY=off  SenseAlphaZ=off  SenseQDDot=off  SenseRDDot=off  SenseX=on  SenseY=on  SenseZ=on  SenseRad=off  SenseAzim=off  SenseDist=off  SenseInc=off  SenseXDot=off  SenseYDot=off  SenseZDot=off  SenseRadDot=off  SenseAzimDot=off  SenseDistDot=off  SenseIncDot=off  SenseXDDot=off  SenseYDDot=off  SenseZDDot=off  SenseRadDDot=off  SenseAzimDDot=off  SenseDistDDot=off  SenseIncDDot=off
  Transport Delay : TransportDelay  DelayTime=1e-6
  Transport Delay1 : TransportDelay  DelayTime=1e-6
  Transport Delay2 : TransportDelay  DelayTime=1e-6
  Variable Cylindrical Solid : sm_lib/Body Elements/Variable Mass/Variable Cylindrical Solid  LengthType=ProvidedByInput  Length=1  LengthUnits=m  RadiusType=Constant  Radius=ligament_radius  RadiusUnits=mm  MassType=CalculateFromGeometry  InitialMassType=Specified  InitialMass=1  InitialMassUnits=kg  Density=0.1  DensityUnits=kg/m^3  SenseRadius=off  SenseLength=off  SenseMass=off  SenseCenterOfMass=off  SenseInertiaMatrix=off  GraphicType=FromGeometry  MarkerShape=Sphere  MarkerSize=10  GraphicVisPropType=SimpleVisualProperties  GraphicDiffuseColor=ISL_color  GraphicSpecularColor=[0.5 0.5 0.5 1.0]  GraphicAmbientColor=[0.15 0.15 0.15 1.0]  GraphicEmissiveColor=[0.0 0.0 0.0 1.0]  GraphicShininess=75  GraphicOpacity=1.0
  MuscleEnd1 : PMIOPort  Side=Right
  MuscleEnd2 : PMIOPort  Port=2  Side=Right
  R : PMIOPort  Port=3  Side=Right
  wires:
  Constant1/1 -> Simulink-PS Converter9/3, Simulink-PS Converter10/3, Simulink-PS Converter11/3
  Constant/1 -> Simulink-PS Converter9/2, Simulink-PS Converter10/2, Simulink-PS Converter11/2
  MATLAB Function2/1(length) -> Simulink-PS Converter/1
  PS-Simulink Converter6/1 -> MATLAB Function2/2(y1)
  PS-Simulink Converter12/1 -> MATLAB Function2/5(y2)
  Transport Delay2/1 -> Simulink-PS Converter11/1
  MATLAB Function2/2(Rx) -> Transport Delay1/1
  MATLAB Function2/3(Ry) -> Transport Delay/1
  PS-Simulink Converter/1 -> MATLAB Function2/1(x1)
  PS-Simulink Converter13/1 -> MATLAB Function2/6(z2)
  Transport Delay1/1 -> Simulink-PS Converter9/1
  PS-Simulink Converter11/1 -> MATLAB Function2/4(x2)
  MATLAB Function2/4(Rz) -> Transport Delay2/1
  Transport Delay/1 -> Simulink-PS Converter10/1
  PS-Simulink Converter7/1 -> MATLAB Function2/3(z1)
  connections:
  MuscleEnd2/RConn1 -- Transform Sensor1/RConn1
  Simulink-PS Converter/RConn1 -- Variable Cylindrical Solid/LConn1
  Transform Sensor1/RConn3 -- PS-Simulink Converter12/LConn1
  Transform Sensor1/LConn1 -- R/RConn1 -- Transform Sensor/LConn1
  Transform Sensor1/RConn4 -- PS-Simulink Converter13/LConn1
  Transform Sensor/RConn2 -- PS-Simulink Converter/LConn1
  Transform Sensor/RConn3 -- PS-Simulink Converter6/LConn1
  Transform Sensor/RConn1 -- MuscleEnd1/RConn1 -- Gimbal Joint/LConn1
  Transform Sensor1/RConn2 -- PS-Simulink Converter11/LConn1
  Gimbal Joint/RConn1 -- Variable Cylindrical Solid/RConn1
  Simulink-PS Converter11/RConn1 -- Gimbal Joint/LConn4
  Simulink-PS Converter10/RConn1 -- Gimbal Joint/LConn3
  Transform Sensor/RConn4 -- PS-Simulink Converter7/LConn1
  Simulink-PS Converter9/RConn1 -- Gimbal Joint/LConn2

== system Main_C0_C3/Interspinous Ligaments/ISL Visualization/Ligament2 ==
  Constant : Constant  Value=0
  Constant1 : Constant  Value=0
  Gimbal Joint : sm_lib/Joints/Gimbal Joint  JointMode=Normal  SenseConstraintForce=off  SenseConstraintForceX=off  SenseConstraintForceY=off  SenseConstraintForceZ=off  SenseConstraintTorque=off  SenseConstraintTorqueX=off  SenseConstraintTorqueY=off  SenseConstraintTorqueZ=off  SenseTotalForce=off  SenseTotalForceX=off  SenseTotalForceY=off  SenseTotalForceZ=off  SenseTotalTorque=off  SenseTotalTorqueX=off  SenseTotalTorqueY=off  SenseTotalTorqueZ=off  CompositeWrenchDir=FollowerOnBase  CompositeWrenchFrame=BaseFrame  RxEquilibriumPosition=0  RxEquilibriumPositionUnits=deg  RxSpringStiffness=0  RxSpringStiffnessUnits=N*m/deg  RxDampingCoefficient=0  RxDampingCoefficientUnits=N*m/(deg/s)  RxTorqueActuationMode=ComputedTorque  RxMotionActuationMode=InputMotion  RxSensePosition=off  RxSenseVelocity=off  RxSenseAcceleration=off  RxSenseTorqueForce=off  RxSenseLowerLimitTorqueForce=off  RxSenseUpperLimitTorqueForce=off  RxLowerLimitSpecify=off  RxLowerLimitBound=-90  RxLowerLimitBoundUnits=deg  RxLowerLimitStiffness=1e4  RxLowerLimitStiffnessUnits=N*m/deg  RxLowerLimitDamping=10  RxLowerLimitDampingUnits=N*m/(deg/s)  RxLowerLimitTransitionRegionWidth=0.1  RxLowerLimitTransitionRegionWidthUnits=deg  RxUpperLimitSpecify=off  RxUpperLimitBound=90  RxUpperLimitBoundUnits=deg  RxUpperLimitStiffness=1e4  RxUpperLimitStiffnessUnits=N*m/deg  RxUpperLimitDamping=10  RxUpperLimitDampingUnits=N*m/(deg/s)  RxUpperLimitTransitionRegionWidth=0.1  RxUpperLimitTransitionRegionWidthUnits=deg  RxPositionTargetSpecify=off  RxPositionTargetPriority=High  RxPositionTargetValue=0  RxPositionTargetValueUnits=deg  RxVelocityTargetSpecify=off  RxVelocityTargetPriority=High  RxVelocityTargetValue=0  RxVelocityTargetValueUnits=deg/s  RyEquilibriumPosition=0  RyEquilibriumPositionUnits=deg  RySpringStiffness=0  RySpringStiffnessUnits=N*m/deg  RyDampingCoefficient=0  RyDampingCoefficientUnits=N*m/(deg/s)  RyTorqueActuationMode=ComputedTorque  RyMotionActuationMode=InputMotion  RySensePosition=off  RySenseVelocity=off  RySenseAcceleration=off  RySenseTorqueForce=off  RySenseLowerLimitTorqueForce=off  RySenseUpperLimitTorqueForce=off  RyLowerLimitSpecify=off  RyLowerLimitBound=-90  RyLowerLimitBoundUnits=deg  RyLowerLimitStiffness=1e4  RyLowerLimitStiffnessUnits=N*m/deg  RyLowerLimitDamping=10  RyLowerLimitDampingUnits=N*m/(deg/s)  RyLowerLimitTransitionRegionWidth=0.1  RyLowerLimitTransitionRegionWidthUnits=deg  RyUpperLimitSpecify=off  RyUpperLimitBound=90  RyUpperLimitBoundUnits=deg  RyUpperLimitStiffness=1e4  RyUpperLimitStiffnessUnits=N*m/deg  RyUpperLimitDamping=10  RyUpperLimitDampingUnits=N*m/(deg/s)  RyUpperLimitTransitionRegionWidth=0.1  RyUpperLimitTransitionRegionWidthUnits=deg  RyPositionTargetSpecify=off  RyPositionTargetPriority=High  RyPositionTargetValue=0  RyPositionTargetValueUnits=deg  RyVelocityTargetSpecify=off  RyVelocityTargetPriority=High  RyVelocityTargetValue=0  RyVelocityTargetValueUnits=deg/s  RzEquilibriumPosition=0  RzEquilibriumPositionUnits=deg  RzSpringStiffness=0  RzSpringStiffnessUnits=N*m/deg  RzDampingCoefficient=0  RzDampingCoefficientUnits=N*m/(deg/s)  RzTorqueActuationMode=ComputedTorque  RzMotionActuationMode=InputMotion  RzSensePosition=off  RzSenseVelocity=off  RzSenseAcceleration=off  RzSenseTorqueForce=off  RzSenseLowerLimitTorqueForce=off  RzSenseUpperLimitTorqueForce=off  RzLowerLimitSpecify=off  RzLowerLimitBound=-90  RzLowerLimitBoundUnits=deg  RzLowerLimitStiffness=1e4  RzLowerLimitStiffnessUnits=N*m/deg  RzLowerLimitDamping=10  RzLowerLimitDampingUnits=N*m/(deg/s)  RzLowerLimitTransitionRegionWidth=0.1  RzLowerLimitTransitionRegionWidthUnits=deg  RzUpperLimitSpecify=off  RzUpperLimitBound=90  RzUpperLimitBoundUnits=deg  RzUpperLimitStiffness=1e4  RzUpperLimitStiffnessUnits=N*m/deg  RzUpperLimitDamping=10  RzUpperLimitDampingUnits=N*m/(deg/s)  RzUpperLimitTransitionRegionWidth=0.1  RzUpperLimitTransitionRegionWidthUnits=deg  RzPositionTargetSpecify=off  RzPositionTargetPriority=High  RzPositionTargetValue=0  RzPositionTargetValueUnits=deg  RzVelocityTargetSpecify=off  RzVelocityTargetPriority=High  RzVelocityTargetValue=0  RzVelocityTargetValueUnits=deg/s
  MATLAB Function2 : MATLAB Function  TreatAsAtomicUnit=on
  PS-Simulink Converter{,6..7,11..13} (6 alike) : nesl_utility/PS-Simulink Converter  PhysicalDomain=network_engine_domain  SubClassName=ps_output  LeftPortType=input  RightPortType=output  PseudoPeriodic=off  Frequencies=[]  VectorFormat=inherit  Unit=inherit  AffineConversion=off
  Simulink-PS Converter : nesl_utility/Simulink-PS Converter  PhysicalDomain=network_engine_domain  SubClassName=ps_input  LeftPortType=input  RightPortType=output  PseudoPeriodic=off  Frequencies=[]  NoiseDistribution=none  NoiseParameters=[]  Unit=m  AffineConversion=off  FilteringAndDerivatives=provide  SimscapeFilterOrder=1  InputFilterTimeConstant=0.001  UdotUserProvided=0
  Simulink-PS Converter10 : nesl_utility/Simulink-PS Converter  PhysicalDomain=network_engine_domain  SubClassName=ps_input  LeftPortType=input  RightPortType=output  PseudoPeriodic=off  Frequencies=[]  NoiseDistribution=none  NoiseParameters=[]  Unit=1  AffineConversion=off  FilteringAndDerivatives=provide  SimscapeFilterOrder=2  InputFilterTimeConstant=0.001  UdotUserProvided=2
  Simulink-PS Converter11 : nesl_utility/Simulink-PS Converter  PhysicalDomain=network_engine_domain  SubClassName=ps_input  LeftPortType=input  RightPortType=output  PseudoPeriodic=off  Frequencies=[]  NoiseDistribution=none  NoiseParameters=[]  Unit=1  AffineConversion=off  FilteringAndDerivatives=provide  SimscapeFilterOrder=2  InputFilterTimeConstant=0.001  UdotUserProvided=2
  Simulink-PS Converter9 : nesl_utility/Simulink-PS Converter  PhysicalDomain=network_engine_domain  SubClassName=ps_input  LeftPortType=input  RightPortType=output  PseudoPeriodic=off  Frequencies=[]  NoiseDistribution=none  NoiseParameters=[]  Unit=1  AffineConversion=on  FilteringAndDerivatives=provide  SimscapeFilterOrder=2  InputFilterTimeConstant=0.1  UdotUserProvided=2
  Transform Sensor : sm_lib/Frames and Transforms/Transform Sensor  MeasurementFrame=Base  RotationSequence=XYZ  SenseAngle=off  SenseAxis=off  SenseQ=off  SenseR=off  SenseRotationSequence=off  SenseOmegaX=off  SenseOmegaY=off  SenseOmegaZ=off  SenseQDot=off  SenseRDot=off  SenseRotationSequenceDot=off  SenseAlphaX=off  SenseAlphaY=off  SenseAlphaZ=off  SenseQDDot=off  SenseRDDot=off  SenseX=on  SenseY=on  SenseZ=on  SenseRad=off  SenseAzim=off  SenseDist=off  SenseInc=off  SenseXDot=off  SenseYDot=off  SenseZDot=off  SenseRadDot=off  SenseAzimDot=off  SenseDistDot=off  SenseIncDot=off  SenseXDDot=off  SenseYDDot=off  SenseZDDot=off  SenseRadDDot=off  SenseAzimDDot=off  SenseDistDDot=off  SenseIncDDot=off
  Transform Sensor1 : sm_lib/Frames and Transforms/Transform Sensor  MeasurementFrame=Base  RotationSequence=XYZ  SenseAngle=off  SenseAxis=off  SenseQ=off  SenseR=off  SenseRotationSequence=off  SenseOmegaX=off  SenseOmegaY=off  SenseOmegaZ=off  SenseQDot=off  SenseRDot=off  SenseRotationSequenceDot=off  SenseAlphaX=off  SenseAlphaY=off  SenseAlphaZ=off  SenseQDDot=off  SenseRDDot=off  SenseX=on  SenseY=on  SenseZ=on  SenseRad=off  SenseAzim=off  SenseDist=off  SenseInc=off  SenseXDot=off  SenseYDot=off  SenseZDot=off  SenseRadDot=off  SenseAzimDot=off  SenseDistDot=off  SenseIncDot=off  SenseXDDot=off  SenseYDDot=off  SenseZDDot=off  SenseRadDDot=off  SenseAzimDDot=off  SenseDistDDot=off  SenseIncDDot=off
  Transport Delay : TransportDelay  DelayTime=1e-6
  Transport Delay1 : TransportDelay  DelayTime=1e-6
  Transport Delay2 : TransportDelay  DelayTime=1e-6
  Variable Cylindrical Solid : sm_lib/Body Elements/Variable Mass/Variable Cylindrical Solid  LengthType=ProvidedByInput  Length=1  LengthUnits=m  RadiusType=Constant  Radius=ligament_radius  RadiusUnits=mm  MassType=CalculateFromGeometry  InitialMassType=Specified  InitialMass=1  InitialMassUnits=kg  Density=0.1  DensityUnits=kg/m^3  SenseRadius=off  SenseLength=off  SenseMass=off  SenseCenterOfMass=off  SenseInertiaMatrix=off  GraphicType=FromGeometry  MarkerShape=Sphere  MarkerSize=10  GraphicVisPropType=SimpleVisualProperties  GraphicDiffuseColor=ISL_color  GraphicSpecularColor=[0.5 0.5 0.5 1.0]  GraphicAmbientColor=[0.15 0.15 0.15 1.0]  GraphicEmissiveColor=[0.0 0.0 0.0 1.0]  GraphicShininess=75  GraphicOpacity=1.0
  MuscleEnd1 : PMIOPort  Side=Right
  MuscleEnd2 : PMIOPort  Port=2  Side=Right
  R : PMIOPort  Port=3  Side=Right
  wires:
  Constant1/1 -> Simulink-PS Converter9/3, Simulink-PS Converter10/3, Simulink-PS Converter11/3
  Constant/1 -> Simulink-PS Converter9/2, Simulink-PS Converter10/2, Simulink-PS Converter11/2
  MATLAB Function2/1(length) -> Simulink-PS Converter/1
  PS-Simulink Converter6/1 -> MATLAB Function2/2(y1)
  PS-Simulink Converter12/1 -> MATLAB Function2/5(y2)
  Transport Delay2/1 -> Simulink-PS Converter11/1
  MATLAB Function2/2(Rx) -> Transport Delay1/1
  MATLAB Function2/3(Ry) -> Transport Delay/1
  PS-Simulink Converter/1 -> MATLAB Function2/1(x1)
  PS-Simulink Converter13/1 -> MATLAB Function2/6(z2)
  Transport Delay1/1 -> Simulink-PS Converter9/1
  PS-Simulink Converter11/1 -> MATLAB Function2/4(x2)
  MATLAB Function2/4(Rz) -> Transport Delay2/1
  Transport Delay/1 -> Simulink-PS Converter10/1
  PS-Simulink Converter7/1 -> MATLAB Function2/3(z1)
  connections:
  MuscleEnd2/RConn1 -- Transform Sensor1/RConn1
  Simulink-PS Converter/RConn1 -- Variable Cylindrical Solid/LConn1
  Transform Sensor1/RConn3 -- PS-Simulink Converter12/LConn1
  Transform Sensor1/LConn1 -- R/RConn1 -- Transform Sensor/LConn1
  Transform Sensor1/RConn4 -- PS-Simulink Converter13/LConn1
  Transform Sensor/RConn2 -- PS-Simulink Converter/LConn1
  Transform Sensor/RConn3 -- PS-Simulink Converter6/LConn1
  Transform Sensor/RConn1 -- MuscleEnd1/RConn1 -- Gimbal Joint/LConn1
  Transform Sensor1/RConn2 -- PS-Simulink Converter11/LConn1
  Gimbal Joint/RConn1 -- Variable Cylindrical Solid/RConn1
  Simulink-PS Converter11/RConn1 -- Gimbal Joint/LConn4
  Simulink-PS Converter10/RConn1 -- Gimbal Joint/LConn3
  Transform Sensor/RConn4 -- PS-Simulink Converter7/LConn1
  Simulink-PS Converter9/RConn1 -- Gimbal Joint/LConn2
